simulink model "positive_and_negative_edge_detection"  (R2021a)
settings: Solver=VariableStepAuto  StartTime=0.0  StopTime=10.0  RelTol=1e-3
libraries: simulink_extras x4
settings Model: Creator=DELL  LastModifiedBy=DELL

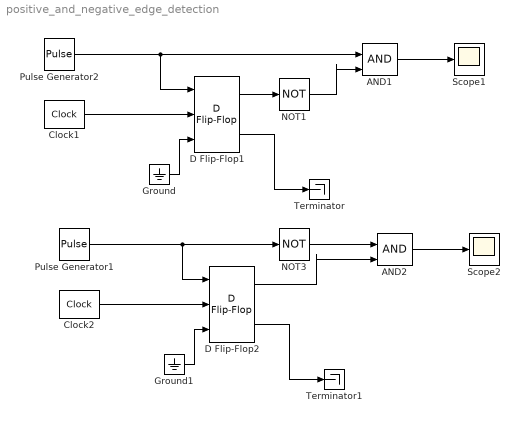
== system positive_and_negative_edge_detection ==
  AND1 : Logic  IconShape=distinctive  AllPortsSameDT=off  OutDataTypeStr=boolean
  AND2 : Logic  IconShape=distinctive  AllPortsSameDT=off  OutDataTypeStr=boolean
  Clock1 : simulink_extras/Flip Flops/Clock  period=1
  Clock2 : simulink_extras/Flip Flops/Clock  period=1
  D Flip-Flop1 : simulink_extras/Flip Flops/D Flip-Flop
  D Flip-Flop2 : simulink_extras/Flip Flops/D Flip-Flop
  Ground : Ground
  Ground1 : Ground
  NOT1 : Logic  Operator=NOT  IconShape=distinctive  AllPortsSameDT=off  OutDataTypeStr=boolean
  NOT3 : Logic  Operator=NOT  IconShape=distinctive  AllPortsSameDT=off  OutDataTypeStr=boolean
  Pulse Generator1 : DiscretePulseGenerator  PulseType=Time based  Period=1  PulseWidth=5
  Pulse Generator2 : DiscretePulseGenerator  PulseType=Time based  Period=1  PulseWidth=5
  Scope1 : Scope
  Scope2 : Scope
  Terminator : Terminator
  Terminator1 : Terminator
  wires:
  Clock1/1 -> D Flip-Flop1/2
  Pulse Generator2/1 -> D Flip-Flop1/1, AND1/1
  D Flip-Flop1/1 -> NOT1/1
  NOT1/1 -> AND1/2
  AND1/1 -> Scope1/1
  Ground/1 -> D Flip-Flop1/3
  D Flip-Flop1/2 -> Terminator/1
  Pulse Generator1/1 -> NOT3/1, D Flip-Flop2/1
  Ground1/1 -> D Flip-Flop2/3
  Clock2/1 -> D Flip-Flop2/2
  D Flip-Flop2/2 -> Terminator1/1
  AND2/1 -> Scope2/1
  D Flip-Flop2/1 -> AND2/2
  NOT3/1 -> AND2/1
